simulink model "rowstan"  (Simulink 8.4)
settings: Solver=ode45  StartTime=0.0  StopTime=Stime  RelTol=1e-3
values from neighbouring files (symbols this model uses):
  A = [(-Kw-crf0)/Cvw, crf0/Cvw; crf0/Cvp, (-Kp-crf0)/Cvp]    [awd.m]
  B = [1/Cvw, Kw/Cvw; 0, Kp/Cvp]    [awd.m]
  C = [1, 0; 0, 1]    [awd.m]
  D = [0, 0; 0, 0]    [awd.m]
  qg0 = 6000    [awd.m]
  qg0t = 60    [awd.m]
  qgInit = 0    [awd.m]
  Tp0 = Twew0*0.35    [awd.m]
  Twew0 = input('Jaka jest temperatura wewnątrz (parter)? [*C] : ')    [awd.m]
  Tzew0 = input('Jaka temperatura jest na zewnątrz? [*C] : ')    [awd.m]
  Tzew1 = input('Jaka będzie temperatura na zewnątrz za godzinę? [*C] : ')    [awd.m]
undefined symbols (not defined in the file or in its folder): qgPower
libraries: simulink x2
settings Model: Creator=kamil  LastModifiedBy=Kamil
settings DebuggingCC: FcnCallInpInsideContextMsg=EnableAllAsWarning
settings GRTTargetCC: CombineOutputUpdateFcns=on  GRTInterface=off

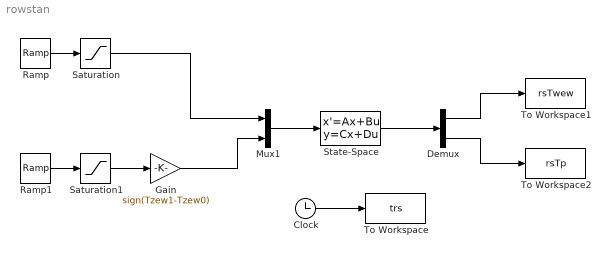
== system rowstan ==
  Clock : Clock
  Demux : Demux  Outputs=2
  Gain : Gain  Gain=sign(Tzew1-Tzew0)
  Mux1 : Mux  Inputs=2
  Ramp : simulink/Sources/Ramp  slope=qg0/qg0t  start=0  X0=qgInit
  Ramp1 : simulink/Sources/Ramp  slope=abs(Tzew1-Tzew0)/3600  start=0  X0=abs(Tzew0)
  Saturation : Saturate  UpperLimit=qg0*qgPower  LowerLimit=0
  Saturation1 : Saturate  UpperLimit=max(abs(Tzew0),abs(Tzew1))  LowerLimit=0
  State-Space : StateSpace  A=A  B=B  C=C  D=D  X0=[Twew0 Tp0]  ContinuousStateAttributes='temperatura'
  To Workspace : ToWorkspace  VariableName=trs  SampleTime=-1
  To Workspace1 : ToWorkspace  VariableName=rsTwew  SampleTime=-1
  To Workspace2 : ToWorkspace  VariableName=rsTp  SampleTime=-1
  wires:
  Mux1/1 -> State-Space/1
  State-Space/1 -> Demux/1
  Demux/1 -> To Workspace1/1
  Demux/2 -> To Workspace2/1
  Clock/1 -> To Workspace/1
  Ramp/1 -> Saturation/1
  Saturation/1 -> Mux1/1
  Ramp1/1 -> Saturation1/1
  Saturation1/1 -> Gain/1
  Gain/1 -> Mux1/2
